simulink model "Controller"  (R2024b)
settings: Solver=ode4  StartTime=0.0  StopTime=inf  FixedStep=.01  RelTol=1e-3  EnableMultiTasking=on
model workspace (MAT data in the model file):
  Active_Scenario_Index = 1
  BattChrgMax = -105500
  BattDischrgMax = 211000
  BattTempInit = 25
  Battery.SOC_LUT = [0.01 0.02 0.03 0.04 0.05 0.06 0.07 0.08 0.09 0.1 0.11 0.12 0.13 0.14 0.15 0.16 0.17 0.18 0.19 0.2 0.21 0.22 0.23 0.24 0.25 0.26 0.27 0.28 0.29 0.3 0.31 0.32 0.33 0.34 0.35 0.36 0.37 0.38 0.39 0.4 0.41 0.42 0.43 0.44 0.45 0.46 0.47 0.48 0.49 0.5 0.51 0.52 0.53 0.54 0.55 0.56 0.57 0.58 0.59 0.6 0.61 0.62 0.63 0.64 0.65 0.66 0.67 0.68 0.69 0.7 0.71 0.72 0.73 0.74 0.75 0.76 0.77 0.78 0.79 0.8 0.81 0.82 0.83 0.84 0.85 0.86 0.87 0.88 0.89 0.9 0.91 0.92 0.93 0.94 0.95 0.96 0.97 0.98 0.99 1]
  Battery.Temperature_LUT = [-10 0 25 40]
  Battery.Capacity_LUT = [4.04528301887 4.19622641509 4.8 4.73962264151]
  Battery.Em_LUT = [2.67308083891 2.74411674384 2.80408613071 2.86247711994 2.90851059763 2.94904306488 2.9829846776 3.01467102589 3.04031502638 3.06256828113 3.08180972392 3.09994219643 ... (400 elements, 100x4)]
  Battery.R0_LUT = [0.0569026752707 0.0575506938969 0.0576730924021 0.0575627404981 0.0573787336615 0.0571931123197 0.0568199985482 0.056411926464 0.0561974340667 0.0560805640861 0.0557640899305 0.055275807865 ... (400 elements, 100x4)]
  Battery.R1_LUT = [0.0035 0.0035 0.0035 0.0035 0.0035 0.0035 0.0035 0.0035 0.0035 0.0035 0.0035 0.0035 ... (400 elements, 100x4)]
  Battery.C1_LUT = [5000 5000 5000 5000 5000 5000 5000 5000 5000 5000 5000 5000 ... (400 elements, 100x4)]
  Battery.Mass = 0.047
  Battery.ThermalMass = 44
  Battery.R_bleed = 20
  Battery.h_conv = 5
  Battery.cell_area = 0.0037
  Battery.TempInit = 25
  Battery.SOCInit = 0.75
  Battery.Model = 'panasonic ncr18650bd'
  Battery.DischargeCycle_LUT = [1 5 9 13 17 21 25 29 33 37 41 45 49 53 57 61 65 69 73 77 81 85 89 93 97 101 105 109 113 117 121 125 129 133 137 141 145 149 153 157 161 165 169 173 177 181 185 189 193 197 201 205 209 213 217 221 225 229 233 237 241 245 249 253 257 261 265 269 273 277 281 285 289 293 297 301 305 309 313 317]
  Battery.deltaEm_LUT = [0 -0.363115641304 -0.600096647258 -0.689070000839 -0.76773380251 -0.846397604181 -0.926368385458 -0.992711297521 -1.05704974111 -1.12227693902 -1.19018070587 -1.25808447272 -1.31699459748 -1.35876443799 -1.40168267642 -1.44460091485 -1.48751915327 -1.5304373917 -1.57335563013 -1.62198241593 -1.67232184498 -1.71858340023 -1.76179802551 -1.8050126508 -1.84822727608 -1.8917937136 -1.93575272784 -1.97971174208 -2.02367075632 -2.06762977056 -2.11171979109 -2.15588700406 -2.19980020032 -2.24365853098 -2.28751686164 -2.33137519231 -2.37523352297 -2.41909185363 -2.45982559031 -2.49599372373 -2.53216185715 -2.56832999058 -2.604498124 -2.64066625743 -2.67683439085 -2.71300252428 -2.7491706577 -2.78367585394 -2.81632179346 -2.8483348579 -2.88034792233 -2.91236098677 -2.94437405121 -2.97638711564 -3.00840018008 -3.04041324451 -3.07260346059 -3.10359008254 -3.13082308991 -3.15805609728 -3.18528910464 -3.21252211201 -3.23975511938 -3.26698812675 -3.29422113412 -3.32122400938 -3.3463475604 -3.37152613073 -3.39670470105 -3.42188327138 -3.4470618417 -3.47224041203 -3.49938358795 -3.52900276724 -3.55862194653 -3.58824112582 -3.6178603051 -3.64748858268 -3.67711690909 -3.70674523549]
  Battery.deltaCapacity_LUT = [0 -0.860019120059 -1.71332421702 -2.0819400264 -2.45055583577 -2.81917164515 -3.18778745452 -3.48884924257 -3.7808148236 -4.07278040463 -4.36474598566 -4.6567115667 -4.91000721732 -5.08494410056 -5.2598809838 -5.43481786703 -5.60975475027 -5.78469163351 -5.95962851674 -6.13456539998 -6.30950228322 -6.47026795816 -6.62044510558 -6.77062225299 -6.92079940041 -7.07097654783 -7.22115369524 -7.37133084266 -7.52150799007 -7.67168513749 -7.82230984162 -7.97319825819 -8.12408667477 -8.27497509134 -8.42586350792 -8.57675192449 -8.72764034107 -8.87852875764 -9.01789522921 -9.13717923376 -9.25646323831 -9.37574724285 -9.4950312474 -9.61431525195 -9.73359925649 -9.85288326104 -9.97216726558 -10.0914512701 -10.2059878191 -10.3183039593 -10.4306200996 -10.5429362398 -10.65525238 -10.7675685203 -10.8798846605 -10.9922008008 -11.104516941 -11.2125891929 -11.3075699376 -11.4025506823 -11.4975314271 -11.5925121718 -11.6874929166 -11.7824736613 -11.877454406 -11.9716325175 -12.0588579537 -12.1460833899 -12.2333088261 -12.3205342623 -12.4077596986 -12.4949851348 -12.5890165008 -12.6916254178 -12.7942343349 -12.8968432519 -12.999452169 -13.102061086 -13.2046700031 -13.3072789201]
  Battery.cond_thickness = 0.001
  Battery.thermal_conductivity = 205
  BrkPrsMax = 5000000
  CellType = 1
  ChrgLmt_bpt = [1 1 1 1 1 1 1 1 0.7 0.35 0]
  DischrgLmt_bpt = [0 0.35 0.7 1 1 1 1 1 1 1 1]
  MotMapEff = 0
  MotSpd = [0 1600 3200 4477.56 4800 6400 8000 9600 11200 12800 14400 16000]
  MotTrq = [450 450 450 450 419.771162405 314.828371804 251.862697443 209.885581202 179.901926745 157.414185902 139.923720802 125.931348721]
  Ndiff = 9.04
  Np_Module = 31
  Ns_Module = 24
  NumModules = 4
  OverCellVoltageLimit = 4.19999980927
  RegenBrkCutOff = [0 1]
  RegenBrkSpd_bpt = [5 9]
  Rm = 0.15
  SOC_bpt = [0 10 20 30 40 50 60 70 80 90 100]
  T_eff_bp = [0 32.1428571429 64.2857142857 96.4285714286 128.571428571 160.714285714 192.857142857 225 257.142857143 289.285714286 321.428571429 353.571428571 385.714285714 417.857142857 450]
  TestCase = 1
  UnderCellVoltageLimit = 2.5
  disk_abore = 0.05
  efficiency_table = [86.7  86.7  86.7  86.7  86.7  86.7  86.7  86.7  86.7  86.7  86.7  86.7  86.7  86.7  86.7; 86.7  86.7  86.7  86.7  86.7  86.7  86.7  86.7  86.7  86.7  86.7  86.7  86.7  86.7  86.7; 86.7  86.7  91.8  91.8  91.8  91.8  91.8  91.8  91.8  91.8  89.76  89.76  89.76  89.76  89.76; 86.7  86.7  93.84  93.84  93.84  93.84  93.84  93.84  93.84  93.84  93.84  91.8  91.8  91.8  91.8; 86.7  86.7  93.84  93.84  94.86  94.86  94.86  94.86  93.84  93.84  93.84  91.8  91.8  91.8  91.8; 86.7  86.7  94.86  95.88  95.88  95.88  95.88  95.88  95.88  95.88  95.88  95.88  95.88  95.88  95.88; 86.7  86.7  94.86  95.88  95.88  96.9  96.9  96.9  96.9  96.9  96.9  96.9  96.9  96.9  96.9; 86.7  86.7  94.86  95.88  95.88  96.9  96.9  96.9  96.9  96.9  96.9  96.9  96.9  96.9  96.9; 86.7  86.7  94.86  95.88  96.9  96.9  96.9  96.9  96.9  96.9  96.9  96.9  96.9  96.9  96.9; 86.7  86.7  94.86  95.88  96.9  96.9  96.9  96.9  96.9  96.9  96.9  96.9  96.9  96.9  96.9; 86.7  86.7  94.86  95.88  95.88  95.88  95.88  95.88  95.88  95.88  95.88  95.88  95.88  95.88  95.88; 86.7  86.7  91.8  93.84  94.86  94.86  94.86  94.86  94.86  94.86  94.86  94.86  94.86  94.86  94.86]
  mu_kinetic = 0.35
  num_pads = 2
  ts = 0.1
  w_eff_bp = [0 1600 3200 4477.56 4800 6400 8000 9600 11200 12800 14400 16000]
libraries: simulink x2
settings Model: Creator=jungj  LastModifiedBy=jungj

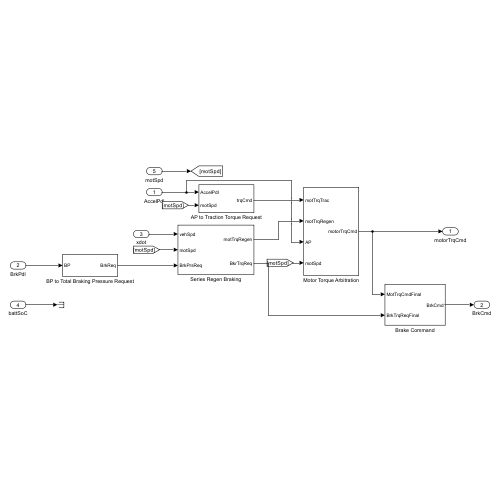
[thumbnail: Simulink's stored preview of the top-level diagram]
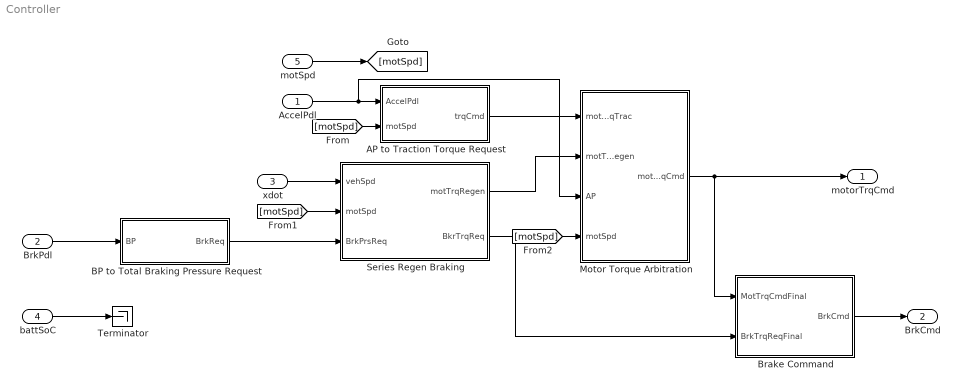
== system Controller ==
  AccelPdl : Inport
  BrkPdl : Inport  Port=2
  xdot : Inport  Port=3
  battSoC : Inport  Port=4
  motSpd : Inport  Port=5
  AP to Traction Torque Request : Subsystem
  BP to Total Braking Pressure Request : Subsystem
  Brake Command : Subsystem
  Motor Torque Arbitration : Subsystem
  Series Regen Braking : Subsystem
  Terminator : Terminator
  motorTrqCmd : Outport
  BrkCmd : Outport  Port=2
  wires:
  motSpd/1 -> [motSpd]
  AccelPdl/1 -> Motor Torque Arbitration/3(AP), AP to Traction Torque Request/1(AccelPdl)
  [motSpd] -> AP to Traction Torque Request/2(motSpd)
  BrkPdl/1 -> BP to Total Braking Pressure Request/1(BP)
  BP to Total Braking Pressure Request/1(BrkReq) -> Series Regen Braking/3(BrkPrsReq)
  [motSpd] -> Series Regen Braking/2(motSpd)
  xdot/1 -> Series Regen Braking/1(vehSpd)
  Brake Command/1(BrkCmd) -> BrkCmd/1
  Motor Torque Arbitration/1(motorTrqCmd) -> Brake Command/1(MotTrqCmdFinal), motorTrqCmd/1
  Series Regen Braking/2(BkrTrqReq) -> Brake Command/2(BrkTrqReqFinal)
  Series Regen Braking/1(motTrqRegen) -> Motor Torque Arbitration/2(motTrqRegen)
  AP to Traction Torque Request/1(trqCmd) -> Motor Torque Arbitration/1(motTrqTrac)
  [motSpd] -> Motor Torque Arbitration/4(motSpd)
  battSoC/1 -> Terminator/1

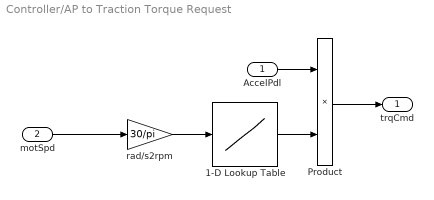
== system Controller/AP to Traction Torque Request ==
  AccelPdl : Inport
  motSpd : Inport  Port=2
  1-D Lookup Table : Lookup_n-D  NumberOfTableDimensions=1  BreakpointsForDimension1=MotSpd  Table=MotTrq  InternalRulePriority=Speed  RndMeth=Simplest
  Product : Product
  rad/s2rpm : Gain  Gain=30/pi
  trqCmd : Outport
  wires:
  motSpd/1 -> rad/s2rpm/1
  rad/s2rpm/1 -> 1-D Lookup Table/1
  1-D Lookup Table/1 -> Product/2
  AccelPdl/1 -> Product/1
  Product/1 -> trqCmd/1

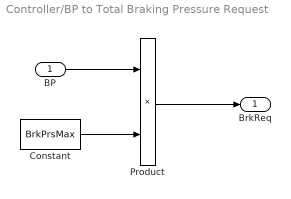
== system Controller/BP to Total Braking Pressure Request ==
  BP : Inport
  Constant : Constant  Value=BrkPrsMax
  Product : Product
  BrkReq : Outport
  wires:
  BP/1 -> Product/1
  Product/1 -> BrkReq/1
  Constant/1 -> Product/2

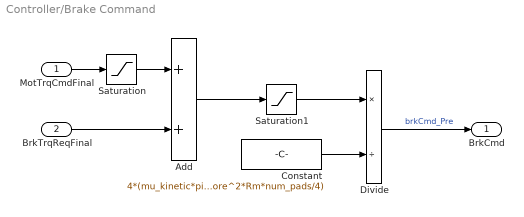
== system Controller/Brake Command ==
  MotTrqCmdFinal : Inport
  BrkTrqReqFinal : Inport  Port=2
  Add : Sum
  Constant : Constant  Value=4*(mu_kinetic*pi*disk_abore^2*Rm*num_pads/4)
  Divide : Product  Inputs=*/
  Saturation : Saturate  UpperLimit=0  LowerLimit=-inf
  Saturation1 : Saturate  UpperLimit=inf  LowerLimit=0
  BrkCmd : Outport
  wires:
  MotTrqCmdFinal/1 -> Saturation/1
  Saturation/1 -> Add/1
  BrkTrqReqFinal/1 -> Add/2
  Add/1 -> Saturation1/1
  Saturation1/1 -> Divide/1
  Constant/1 -> Divide/2
  Divide/1 -> BrkCmd/1  "brkCmd_Pre"

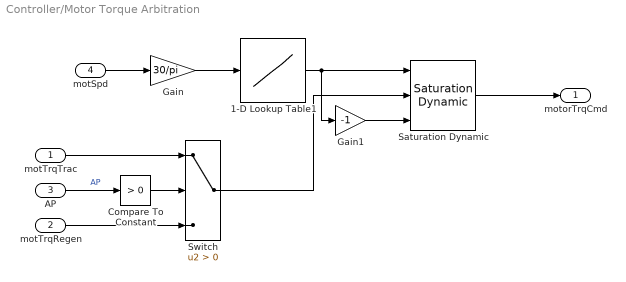
== system Controller/Motor Torque Arbitration ==
  motTrqTrac : Inport
  motTrqRegen : Inport  Port=2
  AP : Inport  Port=3
  motSpd : Inport  Port=4
  1-D Lookup Table1 : Lookup_n-D  NumberOfTableDimensions=1  BreakpointsForDimension1=MotSpd  Table=MotTrq  InternalRulePriority=Speed  RndMeth=Simplest
  Compare To Constant : simulink/Logic and Bit Operations/Compare To Constant  relop=>  const=0  OutDataTypeStr=boolean
  Gain : Gain  Gain=30/pi
  Gain1 : Gain  Gain=-1
  Saturation Dynamic : simulink/Discontinuities/Saturation Dynamic  OutMin=[]  OutMax=[]  OutDataTypeStr=Inherit: Same as second input  OutDataType=fixdt(1, 16)  OutScaling=2^-10  DoSatur=off
  Switch : Switch  Criteria=u2 > Threshold  SaturateOnIntegerOverflow=off  InputSameDT=off
  motorTrqCmd : Outport
  wires:
  AP/1 -> Compare To Constant/1  "AP"
  Compare To Constant/1 -> Switch/2
  motTrqTrac/1 -> Switch/1
  motTrqRegen/1 -> Switch/3
  motSpd/1 -> Gain/1
  Gain/1 -> 1-D Lookup Table1/1
  1-D Lookup Table1/1 -> Gain1/1, Saturation Dynamic/1
  Gain1/1 -> Saturation Dynamic/3
  Switch/1 -> Saturation Dynamic/2
  Saturation Dynamic/1 -> motorTrqCmd/1

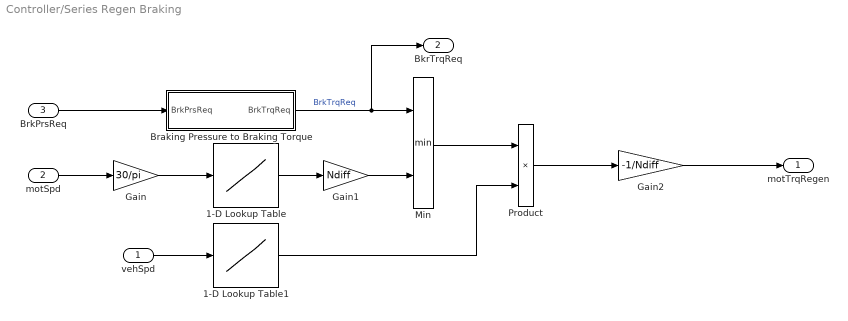
== system Controller/Series Regen Braking ==
  vehSpd : Inport
  motSpd : Inport  Port=2
  BrkPrsReq : Inport  Port=3
  1-D Lookup Table : Lookup_n-D  NumberOfTableDimensions=1  BreakpointsForDimension1=MotSpd  Table=MotTrq  InternalRulePriority=Speed  RndMeth=Simplest
  1-D Lookup Table1 : Lookup_n-D  NumberOfTableDimensions=1  BreakpointsForDimension1=RegenBrkSpd_bpt  Table=RegenBrkCutOff  ExtrapMethod=Clip  UseLastTableValue=on  InternalRulePriority=Speed  RndMeth=Simplest
  Braking Pressure to Braking Torque : Subsystem
  Gain : Gain  Gain=30/pi
  Gain1 : Gain  Gain=Ndiff
  Gain2 : Gain  Gain=-1/Ndiff
  Min : MinMax  Inputs=2
  Product : Product
  motTrqRegen : Outport
  BkrTrqReq : Outport  Port=2
  wires:
  BrkPrsReq/1 -> Braking Pressure to Braking Torque/1(BrkPrsReq)
  Braking Pressure to Braking Torque/1(BrkTrqReq) -> BkrTrqReq/1, Min/1  "BrkTrqReq"
  motSpd/1 -> Gain/1
  Gain/1 -> 1-D Lookup Table/1
  1-D Lookup Table/1 -> Gain1/1
  Gain1/1 -> Min/2
  Min/1 -> Product/1
  vehSpd/1 -> 1-D Lookup Table1/1
  1-D Lookup Table1/1 -> Product/2
  Product/1 -> Gain2/1
  Gain2/1 -> motTrqRegen/1

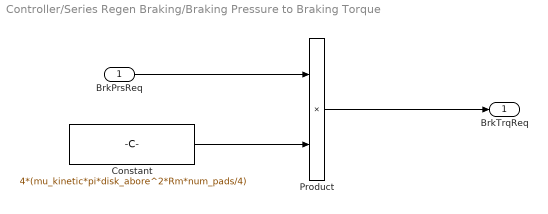
== system Controller/Series Regen Braking/Braking Pressure to Braking Torque ==
  BrkPrsReq : Inport
  Constant : Constant  Value=4*(mu_kinetic*pi*disk_abore^2*Rm*num_pads/4)
  Product : Product
  BrkTrqReq : Outport
  wires:
  BrkPrsReq/1 -> Product/1
  Constant/1 -> Product/2
  Product/1 -> BrkTrqReq/1
